simulink model "cartPole_QFT_mdl"  (R2022b)
settings: Solver=ode4  StartTime=0.0  StopTime=0.5  FixedStep=.001  RelTol=1e-3
undefined symbols (not defined in the file): F_x, G_theta, G_x, sys_theory
settings Model: Creator=mo780715  LastModifiedBy=mo780715

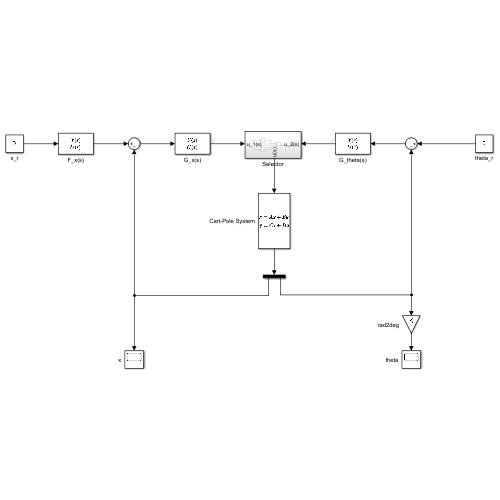
[thumbnail: Simulink's stored preview of the top-level diagram]
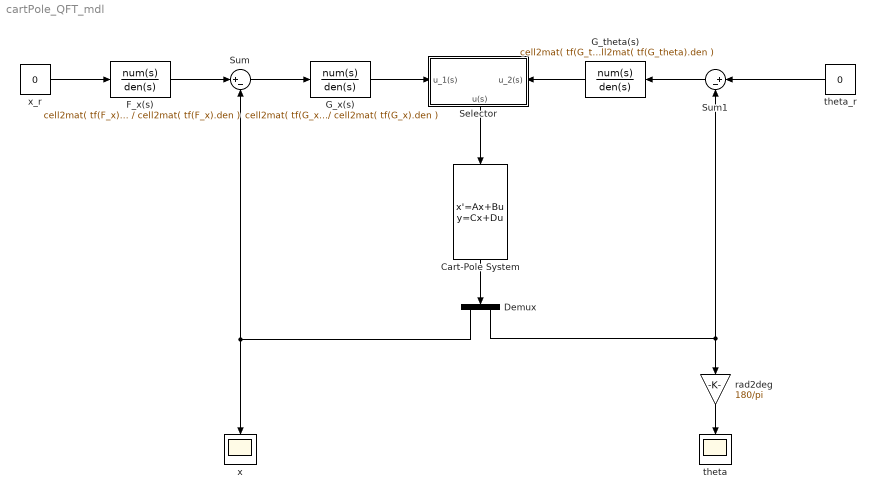
== system cartPole_QFT_mdl ==
  Cart-Pole System : StateSpace  A=sys_theory.A  B=sys_theory.B  C=sys_theory.C  D=sys_theory.D  InitialCondition=[ 0.1; 0; 0*5/180*pi; 0 ]  ContinuousStateAttributes="[\"x\", \"theta\"]"
  Demux : Demux  Outputs=2
  F_x(s) : TransferFcn  Numerator=cell2mat( tf(F_x).num )  Denominator=cell2mat( tf(F_x).den )
  G_theta(s) : TransferFcn  Numerator=cell2mat( tf(G_theta).num )  Denominator=cell2mat( tf(G_theta).den )
  G_x(s) : TransferFcn  Numerator=cell2mat( tf(G_x).num )  Denominator=cell2mat( tf(G_x).den )
  Selector : Subsystem
      settings: PortSchema="{\"entries\":[{\"content\":{\"sides\":[{\"content\":{\"connectorIds\":[\"In1\"]},\"type\":\"ConnectorPlacement.EquallySpacedRectSide\",\"uuid\":\"9fccf0fa-6994-47ef-b322-0771ca16fa7b\"},{\"content\":{\"connectorIds\":[\"In2\"],\"side\":\"RIGHT\"},\"type\":\"ConnectorPlacement.EquallySpacedRectSide\",\"uuid\":\"0dfb01c2-9883-4dd4-8e2a-158419bfdbc9\"},{\"content\":{\"connectorIds\":[],\"side\":\"TOP\"},\"type\":\"ConnectorPlacement.EquallySpacedRectSide\",\"uuid\":\"efb6f21b-551d-43ce-b394-b74fd7f42e11\"},{\"content\":{\"connectorIds\":[\"Out1\"],\"side\":\"BOTTOM\"},\"type\":\"ConnectorPlacement.EquallySpacedRectSide\",\"uuid\":\"ab58611c-27cd-4cec-9152-8cc366650f86\"}]},\"type\":\"ConnectorPlacement.EquallySpacedConnector\",\"uuid\":\"939a8edc-0832-4a1a-a548-ccbb7d5c0e17\"}],\"packageUris\":[\"http://schema.mathworks.com/mf0/Connector/R2020b\"],\"version\":\"1.0\"}"
  Sum : Sum  Inputs=|+-
  Sum1 : Sum  Inputs=|+-
  rad2deg : Gain  Gain=180/pi
  theta : Scope
  theta_r : Constant  Value=0
  x : Scope
  x_r : Constant  Value=0
  wires:
  x_r/1 -> F_x(s)/1
  Cart-Pole System/1 -> Demux/1
  Demux/1 -> Sum/2, x/1
  Demux/2 -> rad2deg/1, Sum1/2
  F_x(s)/1 -> Sum/1
  theta_r/1 -> Sum1/1
  Sum/1 -> G_x(s)/1
  Sum1/1 -> G_theta(s)/1
  G_x(s)/1 -> Selector/1(u_1(s))
  G_theta(s)/1 -> Selector/2(u_2(s))
  Selector/1(u(s)) -> Cart-Pole System/1
  rad2deg/1 -> theta/1

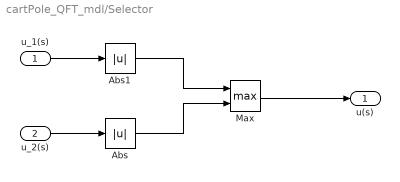
== system cartPole_QFT_mdl/Selector ==
  u_1(s) : Inport
  u_2(s) : Inport  Port=2
  Abs : Abs  SaturateOnIntegerOverflow=off
  Abs1 : Abs  SaturateOnIntegerOverflow=off
  Max : MinMax  Function=max  Inputs=2
  u(s) : Outport
  wires:
  u_2(s)/1 -> Abs/1
  Abs/1 -> Max/2
  u_1(s)/1 -> Abs1/1
  Abs1/1 -> Max/1
  Max/1 -> u(s)/1
